simulink model "Task4Sim"  (R2024b)
settings: Solver=FixedStepDiscrete  StartTime=0.0  StopTime=0.06  FixedStep=1/100000  RelTol=1e-3
libraries: commanapbnd3 x4, dspfdesign x4, dspsrcs4 x4, commchan3 x2
settings Model: Creator=djm23  LastModifiedBy=djm23
settings DataIOCC: ExternalInput=multitoneSignal

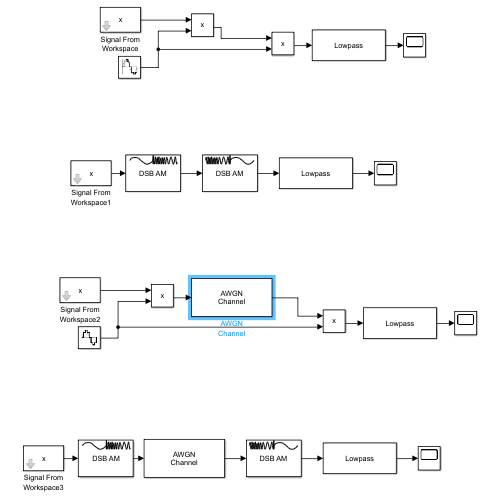
[thumbnail: Simulink's stored preview of the top-level diagram]
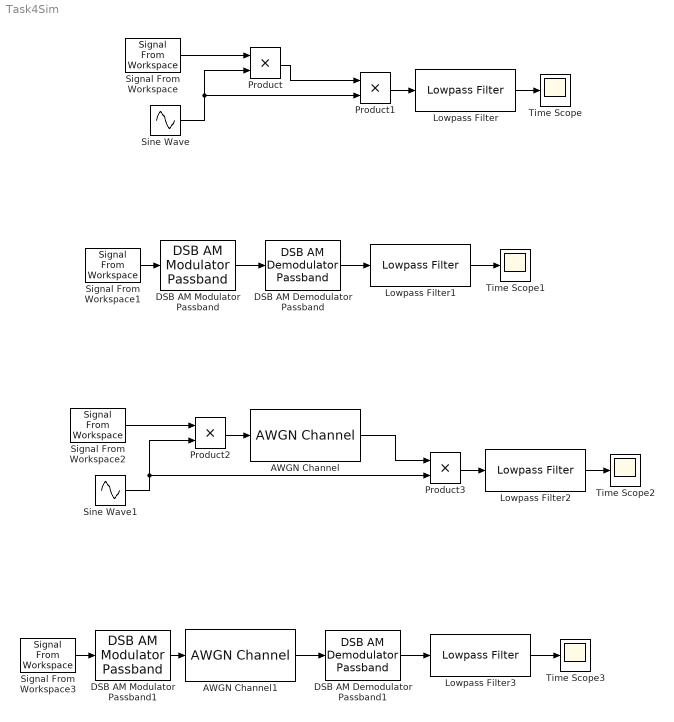
== system Task4Sim ==
  AWGN Channel : commchan3/AWGN Channel  LegacyMode=off  NoiseMethod="Signal to noise ratio  (SNR)"  noiseMode="Signal to noise ratio  (SNR)"  EbNo=10  EsNo=10  SNR=0  BitsPerSymbol=1  SignalPower=1  SamplesPerSymbol=1  SymbolPeriod=1  VarianceSource=Parameter  Variance=1  RandomStream=Global stream  Seed=67  SimulateUsing=Code generation
  AWGN Channel1 : commchan3/AWGN Channel  LegacyMode=off  NoiseMethod="Signal to noise ratio  (SNR)"  noiseMode="Signal to noise ratio  (SNR)"  EbNo=10  EsNo=10  SNR=0  BitsPerSymbol=1  SignalPower=1  SamplesPerSymbol=1  SymbolPeriod=1  VarianceSource=Parameter  Variance=1  RandomStream=Global stream  Seed=67  SimulateUsing=Code generation
  DSB AM Demodulator Passband : commanapbnd3/DSB AM Demodulator Passband  Fc=10000  Ph=0  method=Butterworth  n=4  cf=4000  Rp=0.1  Rs=50  Offset=1
  DSB AM Demodulator Passband1 : commanapbnd3/DSB AM Demodulator Passband  Fc=10000  Ph=0  method=Butterworth  n=4  cf=4000  Rp=0.1  Rs=50  Offset=1
  DSB AM Modulator Passband : commanapbnd3/DSB AM Modulator Passband  Fc=10000  Ph=0  Offset=2
  DSB AM Modulator Passband1 : commanapbnd3/DSB AM Modulator Passband  Fc=10000  Ph=0  Offset=2
  Lowpass Filter{,1..3} (4 alike) : dspfdesign/Lowpass Filter  FilterType=FIR  DesignForMinimumOrder=on  FilterOrder=50  PassbandFrequency=0.3628  StopbandFrequency=0.5442  PassbandRipple=0.1  StopbandAttenuation=80  SampleRateMode=Use normalized frequency (0 to 1)  SampleRate=44100  SimulateUsing=Interpreted execution  roundingMode=Floor  coeffsDataTypeStr=fixdt(1,16)
  Product{,1..3} (4 alike) : Product
  Signal From Workspace{,1..3} (4 alike) : dspsrcs4/Signal From Workspace  X=x  Ts=1/100000  nsamps=1  OutputAfterFinalValue=Setting to zero  ignoreOrWarnInputAndFrameLengths=off  OutputFrames=off
  Sine Wave : Sin  Frequency=2*pi*10000  SampleTime=1/100000
  Sine Wave1 : Sin  Frequency=2*pi*10000  SampleTime=1/100000
  Time Scope{,1..3} (4 alike) : Scope
  wires:
  Signal From Workspace/1 -> Product/1
  Sine Wave/1 -> Product/2, Product1/2
  Product/1 -> Product1/1
  Product1/1 -> Lowpass Filter/1
  Lowpass Filter/1 -> Time Scope/1
  DSB AM Demodulator Passband/1 -> Lowpass Filter1/1
  Lowpass Filter1/1 -> Time Scope1/1
  Signal From Workspace1/1 -> DSB AM Modulator Passband/1
  DSB AM Modulator Passband/1 -> DSB AM Demodulator Passband/1
  Signal From Workspace3/1 -> DSB AM Modulator Passband1/1
  Signal From Workspace2/1 -> Product2/1
  DSB AM Demodulator Passband1/1 -> Lowpass Filter3/1
  Lowpass Filter2/1 -> Time Scope2/1
  Lowpass Filter3/1 -> Time Scope3/1
  Sine Wave1/1 -> Product2/2, Product3/2
  Product3/1 -> Lowpass Filter2/1
  Product2/1 -> AWGN Channel/1
  AWGN Channel/1 -> Product3/1
  DSB AM Modulator Passband1/1 -> AWGN Channel1/1
  AWGN Channel1/1 -> DSB AM Demodulator Passband1/1
